simulink model "prueba1"  (R2021b)
settings: Solver=ode23tb  StartTime=0.0  StopTime=tend  MaxStep=ts  RelTol=1e-3
values from neighbouring files (symbols this model uses):
  tend = 500    [Run_MdE_Research_Report.m]    (also in Run_MdE_Research_Report_con_MR_damper.m; my_script.m)
  ts = 1/fs    (= 0.000666666666667)    [Run_MdE_Research_Report.m]    (also in Run_MdE_Research_Report_con_MR_damper.m; my_script.m)
undefined symbols (not defined in the file or in its folder): D_Gs, N_Gs
libraries: simulink x1, cstblocks x1
settings Model: Creator=luismiguelmartinezgomez  LastModifiedBy=luismiguelmartinezgomez

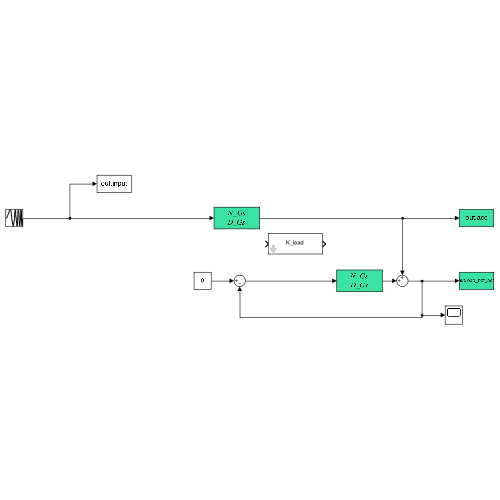
[thumbnail: Simulink's stored preview of the top-level diagram]
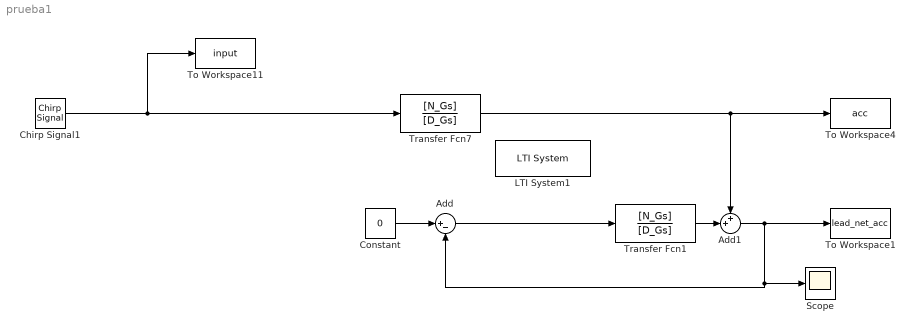
== system prueba1 ==
  Add : Sum  Inputs=|+-
  Add1 : Sum  Inputs=++|
  Chirp Signal1 : simulink/Sources/Chirp Signal  f1=fmin  T=tend  f2=fmax
  Constant : Constant  Value=0
  LTI System1 : cstblocks/LTI System  sys=K_lead  IC=[]
  Scope : Scope
  To Workspace1 : ToWorkspace  VariableName=lead_net_acc  SampleTime=ts
  To Workspace11 : ToWorkspace  VariableName=input  SampleTime=ts
  To Workspace4 : ToWorkspace  VariableName=acc  SampleTime=ts
  Transfer Fcn1 : TransferFcn  Numerator=[N_Gs]  Denominator=[D_Gs]
  Transfer Fcn7 : TransferFcn  Numerator=[N_Gs]  Denominator=[D_Gs]
  wires:
  Transfer Fcn7/1 -> Add1/1, To Workspace4/1
  Add/1 -> Transfer Fcn1/1
  Add1/1 -> To Workspace1/1, Scope/1, Add/2
  Chirp Signal1/1 -> Transfer Fcn7/1, To Workspace11/1
  Transfer Fcn1/1 -> Add1/2
  Constant/1 -> Add/1
